simulink model "shoukong22"  (R2023b)
settings: Solver=FixedStepDiscrete  StartTime=0.0  StopTime=100  FixedStep=1  RelTol=1e-3
settings Model: Creator=54238  LastModifiedBy=54238
settings RTWCC: GPUComputeCapability=5.0

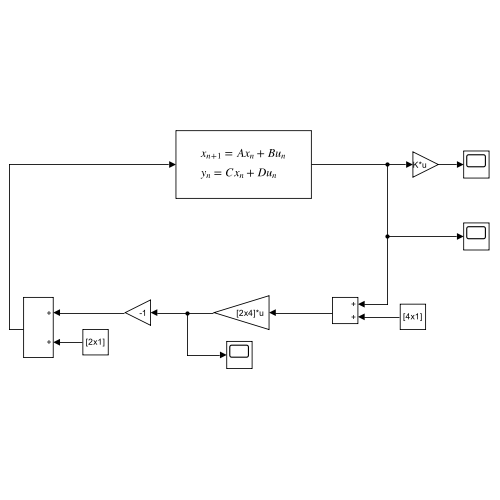
[thumbnail: Simulink's stored preview of the top-level diagram]
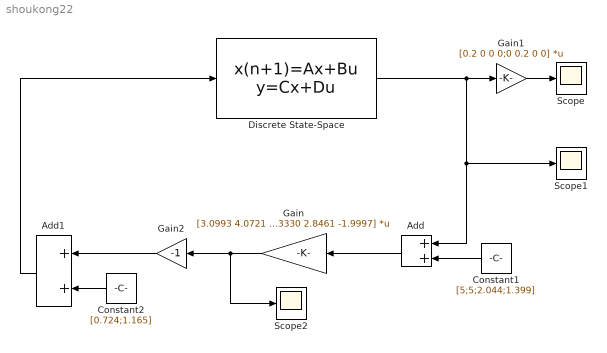
== system shoukong22 ==
  Add : Sum
  Add1 : Sum
  Constant1 : Constant  Value=[5;5;2.044;1.399]  VectorParams1D=off
  Constant2 : Constant  Value=[0.724;1.165]  VectorParams1D=off
  Discrete State-Space : DiscreteStateSpace  A=[0.975 0 0.042 0;0 0.977 0 0.044;0 0 0.958 0;0 0 0 0.956]  B=[0.0515 0.0016;0.0019 0.0447;0 0.0737;0.0850 0]  C=[1 0 0 0;0 1 0 0;0 0 1 0;0 0 0 1]  D=[0 0;0 0;0 0;0 0]  InitialCondition=[10;10;10;10]
  Gain : Gain  Gain=[3.0993 4.0721 -2.0528 2.8417;3.9353 3.3330 2.8461 -1.9997]  Multiplication=Matrix(K*u)
  Gain1 : Gain  Gain=[0.2 0 0 0;0 0.2 0 0]  Multiplication=Matrix(K*u)
  Gain2 : Gain  Gain=-1
  Scope : Scope
  Scope1 : Scope
  Scope2 : Scope
  wires:
  Gain/1 -> Scope2/1, Gain2/1
  Constant1/1 -> Add/2
  Gain2/1 -> Add1/1
  Constant2/1 -> Add1/2
  Add1/1 -> Discrete State-Space/1
  Discrete State-Space/1 -> Scope1/1, Add/1, Gain1/1
  Gain1/1 -> Scope/1
  Add/1 -> Gain/1
